simulink model "Project1_week2_sim"  (R2023b)
settings: Solver=VariableStepAuto  StartTime=0.0  StopTime=25  RelTol=1e-3
values from neighbouring files (symbols this model uses):
  A = [0.0, 100]    [P1_week2_code.m]
  b = [10,0.1]    [P1_week2_code.m]
  freq = [0.1,100]    [P1_week2_code.m]
  J = [100,0.01]    [P1_week2_code.m]
  w_0 = [10.0,0.0]    [P1_week2_code.m]
settings Model: Creator=rahma  LastModifiedBy=rahma

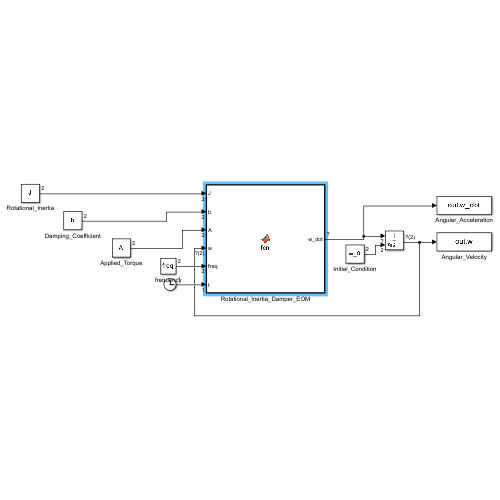
[thumbnail: Simulink's stored preview of the top-level diagram]
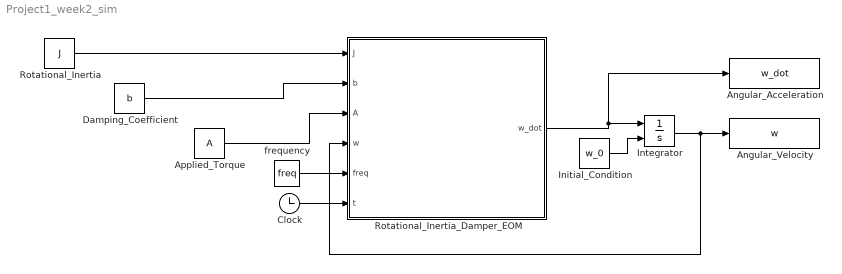
== system Project1_week2_sim ==
  Angular_Acceleration : ToWorkspace  VariableName=w_dot  SaveFormat=Timeseries  SampleTime=-1
  Angular_Velocity : ToWorkspace  VariableName=w  SaveFormat=Timeseries  SampleTime=-1
  Applied_Torque : Constant  Value=A
  Clock : Clock
  Damping_Coefficient : Constant  Value=b
  Initial_Condition : Constant  Value=w_0
  Integrator : Integrator  InitialConditionSource=external
  Rotational_Inertia : Constant  Value=J
  Rotational_Inertia_Damper_EOM : MATLAB Function  TreatAsAtomicUnit=on
  frequency : Constant  Value=freq
  wires:
  frequency/1 -> Rotational_Inertia_Damper_EOM/5(freq)
  Clock/1 -> Rotational_Inertia_Damper_EOM/6(t)
  Initial_Condition/1 -> Integrator/2
  Rotational_Inertia_Damper_EOM/1(w_dot) -> Angular_Acceleration/1, Integrator/1
  Damping_Coefficient/1 -> Rotational_Inertia_Damper_EOM/2(b)
  Applied_Torque/1 -> Rotational_Inertia_Damper_EOM/3(A)
  Rotational_Inertia/1 -> Rotational_Inertia_Damper_EOM/1(J)
  Integrator/1 -> Rotational_Inertia_Damper_EOM/4(w), Angular_Velocity/1

== matlab function Project1_week2_sim/Rotational_Inertia_Damper_EOM ==
  data: J input; w_dot output; b input; A input; w input; freq input; t input
function w_dot = fcn(J, b, A, w, freq, t)
% Recall EOM: J*w_dot = tau_applied - tau_damped
tau_damped = b.*w;
tau = A.*sin(freq.*t)
w_dot = (1/J)*(tau - tau_damped);
end
